simulink model "HIWIN_arm-DESKTOP-VMBR1O2"  (R2022b)
settings: Solver=ode4  StartTime=0  StopTime=1.4435  FixedStep=0.0005  RelTol=1e-3
model workspace (MAT data in the model file):
  Link1_init = 0
  Link2_init = 0
  Link3_init = 0
  Link4_init = 0
  Link5_init = 0
  Link6_init = 0
values from neighbouring files (symbols this model uses):
  b1 = evalin('base','b1')    [Freq_response.m]    (also in Parameters.m = B(1); parameters.mat = 38.5729006482)
  b2 = evalin('base','b2')    [Freq_response.m]    (also in Parameters.m = B(2); parameters.mat = 28.585362141)
  b3 = evalin('base','b3')    [Freq_response.m]    (also in Parameters.m = B(3); parameters.mat = 10.962587304)
  b4 = evalin('base','b4')    [Freq_response.m]    (also in Parameters.m = B(4); parameters.mat = 5.56110095294)
  b5 = evalin('base','b5')    [Freq_response.m]    (also in Parameters.m = B(5); parameters.mat = 1.70954720068)
  b6 = evalin('base','b6')    [Freq_response.m]    (also in Parameters.m = B(6); parameters.mat = 1.09956377442)
  J1 = evalin('base','J1')    [Freq_response.m]    (also in Parameters.m = 2.390528; parameters.mat = 2.390528)
  J2 = evalin('base','J2')    [Freq_response.m]    (also in Parameters.m = 3.0413; parameters.mat = 3.0413)
  J3 = evalin('base','J3')    [Freq_response.m]    (also in Parameters.m = 0.716992; parameters.mat = 0.716992)
  J4 = evalin('base','J4')    [Freq_response.m]    (also in Parameters.m = 0.37850409; parameters.mat = 0.37850409)
  J5 = evalin('base','J5')    [Freq_response.m]    (also in Parameters.m = 0.076544; parameters.mat = 0.076544)
  J6 = evalin('base','J6')    [Freq_response.m]    (also in Parameters.m = 0.03665; parameters.mat = 0.03665)
  Kt1 = evalin('base','Kt1')    [Freq_response.m]    (also in Parameters.m = 0.524; parameters.mat = 0.524)
  Kt2 = evalin('base','Kt2')    [Freq_response.m]    (also in Parameters.m = 0.524; parameters.mat = 0.524)
  Kt3 = evalin('base','Kt3')    [Freq_response.m]    (also in Parameters.m = 0.476; parameters.mat = 0.476)
  Kt4 = evalin('base','Kt4')    [Freq_response.m]    (also in Parameters.m = 0.424; parameters.mat = 0.424)
  Kt5 = evalin('base','Kt5')    [Freq_response.m]    (also in Parameters.m = 0.246; parameters.mat = 0.246)
  Kt6 = evalin('base','Kt6')    [Freq_response.m]    (also in Parameters.m = 0.246; parameters.mat = 0.246)
libraries: slpidlib x38
(part 4 of 4)

== system HIWIN_arm-DESKTOP-VMBR1O2/link test/link6 ==
  In2 : Inport
  In1 : Inport  Port=2
  Integrator : Integrator
  Kp : slpidlib/PID Controller  Controller=PI  Form=Ideal  TimeDomain=Continuous-time  UseExternalTs=off  SampleTime=-1  IntegratorMethod=Forward Euler  FilterMethod=Forward Euler  ControllerParametersSource=internal  P=105.919532331885  I=2.29576855307102  UseKiTs=off  D=0  N=100  UseFilter=on  TunerSelectOption=Transfer Function Based (PID Tuner App)  InitialConditionSource=internal  InitialConditionForIntegrator=0  InitialConditionForFilter=0  DifferentiatorICPrevScaledInput=0  ExternalReset=none  TrackingMode=off  Kt=1  LimitOutput=off  SatLimitsSource=internal  UpperSaturationLimit=inf  LowerSaturationLimit=-inf  LinearizeAsGain=on  AntiWindupMode=none  Kb=1  LimitIntegrator=off  UpperIntegratorSaturationLimit=inf  LowerIntegratorSaturationLimit=-inf  POutMin=[]  POutMax=[]  IOutMin=[]  IOutMax=[]  DOutMin=[]  DOutMax=[]  NOutMin=[]  NOutMax=[]  SumOutMin=[]  SumOutMax=[]  SaturationOutMin=[]  SaturationOutMax=[]  PParamMin=[]  PParamMax=[]  IParamMin=[]  IParamMax=[]  DParamMin=[]  DParamMax=[]  NParamMin=[]  NParamMax=[]  KbParamMin=[]  KbParamMax=[]  KtParamMin=[]  KtParamMax=[]  KbOutMin=[]  KbOutMax=[]  KtOutMin=[]  KtOutMax=[]  IntegratorOutMin=[]  IntegratorOutMax=[]  FilterOutMin=[]  FilterOutMax=[]  SumI1OutMin=[]  SumI1OutMax=[]  SumI2OutMin=[]  SumI2OutMax=[]  SumI3OutMin=[]  SumI3OutMax=[]  SumI4OutMin=[]  SumI4OutMax=[]  SumDOutMin=[]  SumDOutMax=[]  DifferentiatorOutMin=[]  DifferentiatorOutMax=[]  FilterDiffOutCoefMin=[]  FilterDiffOutCoefMax=[]  ReciprocalOutMin=[]  ReciprocalOutMax=[]  SumDenOutMin=[]  SumDenOutMax=[]  SumNumOutMin=[]  SumNumOutMax=[]  DivideOutMin=[]  DivideOutMax=[]  UdiffTsProdOutMin=[]  UdiffTsProdOutMax=[]  NTsProdOutMin=[]  NTsProdOutMax=[]  UintegralTsProdOutMin=[]  UintegralTsProdOutMax=[]  UngainTsProdOutMin=[]  UngainTsProdOutMax=[]  ClampingZeroOutDataTypeStr=Inherit: Inherit via back propagation  ClampingZeroOutMin=[]  ClampingZeroOutMax=[]  FilterDenConstantOutDataTypeStr=Inherit: Inherit via back propagation  FilterDenConstantOutMin=[]  FilterDenConstantOutMax=[]  PCopyOutDataTypeStr=Inherit: Inherit via back propagation  PCopyOutMin=[]  PCopyOutMax=[]  NCopyOutDataTypeStr=Inherit: Inherit via back propagation  NCopyOutMin=[]  NCopyOutMax=[]  IntegratorContinuousStateAttributes=''  IntegratorStateMustResolveToSignalObject=off  IntegratorRTWStateStorageClass=Auto  FilterContinuousStateAttributes=''  FilterStateMustResolveToSignalObject=off  FilterRTWStateStorageClass=Auto  ParallelPVariant=Passthrough  IdealPVariant=InternalParameters  IVariant=InternalParameters  DVariant=Disabled  IntegratorVariant=Continuous  SatVariant=Disabled  AWVariant=Passthrough  PCopyVariant=Disabled  TRVariant=Disabled  FdbkBlocksVariant=Forward  IdealPFdbkVariant=Disabled  SatFdbkVariant=Disabled  DerivativeFilterVariant=Disabled  NVariant=Disabled  NCopyVariant=Disabled_SignalSpec  FilterICVariant=Disabled  IntegratorICVariant=InternalICs  ExternalResetVariant=Disabled  TRSumVariant=Passthrough  SumFdbkVariant=Disabled  SumVariant=Sum_PI  TsampFilterVariant=InternalTs  TsampNgainVariant=Passthrough  TsampIntegralVariant=Passthrough  ExternalSaturationOutDataTypeStr=Inherit: Same as second input
  Kt : Gain  Gain=Kt6
  Kv : slpidlib/PID Controller  Controller=PI  Form=Ideal  TimeDomain=Continuous-time  UseExternalTs=off  SampleTime=-1  IntegratorMethod=Forward Euler  FilterMethod=Forward Euler  ControllerParametersSource=internal  P=21.6698338640267  I=151.095812250567  UseKiTs=off  D=0  N=100  UseFilter=on  TunerSelectOption=Transfer Function Based (PID Tuner App)  InitialConditionSource=internal  InitialConditionForIntegrator=0  InitialConditionForFilter=0  DifferentiatorICPrevScaledInput=0  ExternalReset=none  TrackingMode=off  Kt=1  LimitOutput=off  SatLimitsSource=internal  UpperSaturationLimit=inf  LowerSaturationLimit=-inf  LinearizeAsGain=on  AntiWindupMode=none  Kb=1  LimitIntegrator=off  UpperIntegratorSaturationLimit=inf  LowerIntegratorSaturationLimit=-inf  POutMin=[]  POutMax=[]  IOutMin=[]  IOutMax=[]  DOutMin=[]  DOutMax=[]  NOutMin=[]  NOutMax=[]  SumOutMin=[]  SumOutMax=[]  SaturationOutMin=[]  SaturationOutMax=[]  PParamMin=[]  PParamMax=[]  IParamMin=[]  IParamMax=[]  DParamMin=[]  DParamMax=[]  NParamMin=[]  NParamMax=[]  KbParamMin=[]  KbParamMax=[]  KtParamMin=[]  KtParamMax=[]  KbOutMin=[]  KbOutMax=[]  KtOutMin=[]  KtOutMax=[]  IntegratorOutMin=[]  IntegratorOutMax=[]  FilterOutMin=[]  FilterOutMax=[]  SumI1OutMin=[]  SumI1OutMax=[]  SumI2OutMin=[]  SumI2OutMax=[]  SumI3OutMin=[]  SumI3OutMax=[]  SumI4OutMin=[]  SumI4OutMax=[]  SumDOutMin=[]  SumDOutMax=[]  DifferentiatorOutMin=[]  DifferentiatorOutMax=[]  FilterDiffOutCoefMin=[]  FilterDiffOutCoefMax=[]  ReciprocalOutMin=[]  ReciprocalOutMax=[]  SumDenOutMin=[]  SumDenOutMax=[]  SumNumOutMin=[]  SumNumOutMax=[]  DivideOutMin=[]  DivideOutMax=[]  UdiffTsProdOutMin=[]  UdiffTsProdOutMax=[]  NTsProdOutMin=[]  NTsProdOutMax=[]  UintegralTsProdOutMin=[]  UintegralTsProdOutMax=[]  UngainTsProdOutMin=[]  UngainTsProdOutMax=[]  ClampingZeroOutDataTypeStr=Inherit: Inherit via back propagation  ClampingZeroOutMin=[]  ClampingZeroOutMax=[]  FilterDenConstantOutDataTypeStr=Inherit: Inherit via back propagation  FilterDenConstantOutMin=[]  FilterDenConstantOutMax=[]  PCopyOutDataTypeStr=Inherit: Inherit via back propagation  PCopyOutMin=[]  PCopyOutMax=[]  NCopyOutDataTypeStr=Inherit: Inherit via back propagation  NCopyOutMin=[]  NCopyOutMax=[]  IntegratorContinuousStateAttributes=''  IntegratorStateMustResolveToSignalObject=off  IntegratorRTWStateStorageClass=Auto  FilterContinuousStateAttributes=''  FilterStateMustResolveToSignalObject=off  FilterRTWStateStorageClass=Auto  ParallelPVariant=Passthrough  IdealPVariant=InternalParameters  IVariant=InternalParameters  DVariant=Disabled  IntegratorVariant=Continuous  SatVariant=Disabled  AWVariant=Passthrough  PCopyVariant=Disabled  TRVariant=Disabled  FdbkBlocksVariant=Forward  IdealPFdbkVariant=Disabled  SatFdbkVariant=Disabled  DerivativeFilterVariant=Disabled  NVariant=Disabled  NCopyVariant=Disabled_SignalSpec  FilterICVariant=Disabled  IntegratorICVariant=InternalICs  ExternalResetVariant=Disabled  TRSumVariant=Passthrough  SumFdbkVariant=Disabled  SumVariant=Sum_PI  TsampFilterVariant=InternalTs  TsampNgainVariant=Passthrough  TsampIntegralVariant=Passthrough  ExternalSaturationOutDataTypeStr=Inherit: Same as second input
  Sum2 : Sum  Inputs=|+-
  Sum3 : Sum  Inputs=|+-
  Sum4 : Sum  Inputs=|+-
  Transfer Fcn1 : TransferFcn  Denominator=[J6 b6]
  theta : Outport
  wires:
  Sum2/1 -> Kv/1
  Transfer Fcn1/1 -> Integrator/1, Sum2/2  "theta dot"
  Kv/1 -> Kt/1
  Kt/1 -> Sum4/1  "T"
  Sum4/1 -> Transfer Fcn1/1
  In2/1 -> Sum4/2
  Sum3/1 -> Kp/1
  Kp/1 -> Sum2/1
  In1/1 -> Sum3/1
  Integrator/1 -> Sum3/2, theta/1

== system HIWIN_arm-DESKTOP-VMBR1O2/link test/link6_test ==
  In1 : Inport
  Integrator : Integrator
  Kp : slpidlib/PID Controller  Controller=PI  Form=Ideal  TimeDomain=Continuous-time  UseExternalTs=off  SampleTime=-1  IntegratorMethod=Forward Euler  FilterMethod=Forward Euler  ControllerParametersSource=internal  P=5.27011747503354  I=0.0922424275458122  UseKiTs=off  D=0  N=100  UseFilter=on  TunerSelectOption=Transfer Function Based (PID Tuner App)  InitialConditionSource=internal  InitialConditionForIntegrator=0  InitialConditionForFilter=0  DifferentiatorICPrevScaledInput=0  ExternalReset=none  TrackingMode=off  Kt=1  LimitOutput=off  SatLimitsSource=internal  UpperSaturationLimit=inf  LowerSaturationLimit=-inf  LinearizeAsGain=on  AntiWindupMode=none  Kb=1  LimitIntegrator=off  UpperIntegratorSaturationLimit=inf  LowerIntegratorSaturationLimit=-inf  POutMin=[]  POutMax=[]  IOutMin=[]  IOutMax=[]  DOutMin=[]  DOutMax=[]  NOutMin=[]  NOutMax=[]  SumOutMin=[]  SumOutMax=[]  SaturationOutMin=[]  SaturationOutMax=[]  PParamMin=[]  PParamMax=[]  IParamMin=[]  IParamMax=[]  DParamMin=[]  DParamMax=[]  NParamMin=[]  NParamMax=[]  KbParamMin=[]  KbParamMax=[]  KtParamMin=[]  KtParamMax=[]  KbOutMin=[]  KbOutMax=[]  KtOutMin=[]  KtOutMax=[]  IntegratorOutMin=[]  IntegratorOutMax=[]  FilterOutMin=[]  FilterOutMax=[]  SumI1OutMin=[]  SumI1OutMax=[]  SumI2OutMin=[]  SumI2OutMax=[]  SumI3OutMin=[]  SumI3OutMax=[]  SumI4OutMin=[]  SumI4OutMax=[]  SumDOutMin=[]  SumDOutMax=[]  DifferentiatorOutMin=[]  DifferentiatorOutMax=[]  FilterDiffOutCoefMin=[]  FilterDiffOutCoefMax=[]  ReciprocalOutMin=[]  ReciprocalOutMax=[]  SumDenOutMin=[]  SumDenOutMax=[]  SumNumOutMin=[]  SumNumOutMax=[]  DivideOutMin=[]  DivideOutMax=[]  UdiffTsProdOutMin=[]  UdiffTsProdOutMax=[]  NTsProdOutMin=[]  NTsProdOutMax=[]  UintegralTsProdOutMin=[]  UintegralTsProdOutMax=[]  UngainTsProdOutMin=[]  UngainTsProdOutMax=[]  ClampingZeroOutDataTypeStr=Inherit: Inherit via back propagation  ClampingZeroOutMin=[]  ClampingZeroOutMax=[]  FilterDenConstantOutDataTypeStr=Inherit: Inherit via back propagation  FilterDenConstantOutMin=[]  FilterDenConstantOutMax=[]  PCopyOutDataTypeStr=Inherit: Inherit via back propagation  PCopyOutMin=[]  PCopyOutMax=[]  NCopyOutDataTypeStr=Inherit: Inherit via back propagation  NCopyOutMin=[]  NCopyOutMax=[]  IntegratorContinuousStateAttributes=''  IntegratorStateMustResolveToSignalObject=off  IntegratorRTWStateStorageClass=Auto  FilterContinuousStateAttributes=''  FilterStateMustResolveToSignalObject=off  FilterRTWStateStorageClass=Auto  ParallelPVariant=Passthrough  IdealPVariant=InternalParameters  IVariant=InternalParameters  DVariant=Disabled  IntegratorVariant=Continuous  SatVariant=Disabled  AWVariant=Passthrough  PCopyVariant=Disabled  TRVariant=Disabled  FdbkBlocksVariant=Forward  IdealPFdbkVariant=Disabled  SatFdbkVariant=Disabled  DerivativeFilterVariant=Disabled  NVariant=Disabled  NCopyVariant=Disabled_SignalSpec  FilterICVariant=Disabled  IntegratorICVariant=InternalICs  ExternalResetVariant=Disabled  TRSumVariant=Passthrough  SumFdbkVariant=Disabled  SumVariant=Sum_PI  TsampFilterVariant=InternalTs  TsampNgainVariant=Passthrough  TsampIntegralVariant=Passthrough  ExternalSaturationOutDataTypeStr=Inherit: Same as second input
  Kt : Gain  Gain=Kt6
  Kv : slpidlib/PID Controller  Controller=PI  Form=Ideal  TimeDomain=Continuous-time  UseExternalTs=off  SampleTime=-1  IntegratorMethod=Forward Euler  FilterMethod=Forward Euler  ControllerParametersSource=internal  P=8.61933922965824e-06  I=187982.02415467  UseKiTs=off  D=0  N=100  UseFilter=on  TunerSelectOption=Transfer Function Based (PID Tuner App)  InitialConditionSource=internal  InitialConditionForIntegrator=0  InitialConditionForFilter=0  DifferentiatorICPrevScaledInput=0  ExternalReset=none  TrackingMode=off  Kt=1  LimitOutput=off  SatLimitsSource=internal  UpperSaturationLimit=inf  LowerSaturationLimit=-inf  LinearizeAsGain=on  AntiWindupMode=none  Kb=1  LimitIntegrator=off  UpperIntegratorSaturationLimit=inf  LowerIntegratorSaturationLimit=-inf  POutMin=[]  POutMax=[]  IOutMin=[]  IOutMax=[]  DOutMin=[]  DOutMax=[]  NOutMin=[]  NOutMax=[]  SumOutMin=[]  SumOutMax=[]  SaturationOutMin=[]  SaturationOutMax=[]  PParamMin=[]  PParamMax=[]  IParamMin=[]  IParamMax=[]  DParamMin=[]  DParamMax=[]  NParamMin=[]  NParamMax=[]  KbParamMin=[]  KbParamMax=[]  KtParamMin=[]  KtParamMax=[]  KbOutMin=[]  KbOutMax=[]  KtOutMin=[]  KtOutMax=[]  IntegratorOutMin=[]  IntegratorOutMax=[]  FilterOutMin=[]  FilterOutMax=[]  SumI1OutMin=[]  SumI1OutMax=[]  SumI2OutMin=[]  SumI2OutMax=[]  SumI3OutMin=[]  SumI3OutMax=[]  SumI4OutMin=[]  SumI4OutMax=[]  SumDOutMin=[]  SumDOutMax=[]  DifferentiatorOutMin=[]  DifferentiatorOutMax=[]  FilterDiffOutCoefMin=[]  FilterDiffOutCoefMax=[]  ReciprocalOutMin=[]  ReciprocalOutMax=[]  SumDenOutMin=[]  SumDenOutMax=[]  SumNumOutMin=[]  SumNumOutMax=[]  DivideOutMin=[]  DivideOutMax=[]  UdiffTsProdOutMin=[]  UdiffTsProdOutMax=[]  NTsProdOutMin=[]  NTsProdOutMax=[]  UintegralTsProdOutMin=[]  UintegralTsProdOutMax=[]  UngainTsProdOutMin=[]  UngainTsProdOutMax=[]  ClampingZeroOutDataTypeStr=Inherit: Inherit via back propagation  ClampingZeroOutMin=[]  ClampingZeroOutMax=[]  FilterDenConstantOutDataTypeStr=Inherit: Inherit via back propagation  FilterDenConstantOutMin=[]  FilterDenConstantOutMax=[]  PCopyOutDataTypeStr=Inherit: Inherit via back propagation  PCopyOutMin=[]  PCopyOutMax=[]  NCopyOutDataTypeStr=Inherit: Inherit via back propagation  NCopyOutMin=[]  NCopyOutMax=[]  IntegratorContinuousStateAttributes=''  IntegratorStateMustResolveToSignalObject=off  IntegratorRTWStateStorageClass=Auto  FilterContinuousStateAttributes=''  FilterStateMustResolveToSignalObject=off  FilterRTWStateStorageClass=Auto  ParallelPVariant=Passthrough  IdealPVariant=InternalParameters  IVariant=InternalParameters  DVariant=Disabled  IntegratorVariant=Continuous  SatVariant=Disabled  AWVariant=Passthrough  PCopyVariant=Disabled  TRVariant=Disabled  FdbkBlocksVariant=Forward  IdealPFdbkVariant=Disabled  SatFdbkVariant=Disabled  DerivativeFilterVariant=Disabled  NVariant=Disabled  NCopyVariant=Disabled_SignalSpec  FilterICVariant=Disabled  IntegratorICVariant=InternalICs  ExternalResetVariant=Disabled  TRSumVariant=Passthrough  SumFdbkVariant=Disabled  SumVariant=Sum_PI  TsampFilterVariant=InternalTs  TsampNgainVariant=Passthrough  TsampIntegralVariant=Passthrough  ExternalSaturationOutDataTypeStr=Inherit: Same as second input
  Scope : Scope
  Sum2 : Sum  Inputs=|+-
  Sum3 : Sum  Inputs=|+-
  Transfer Fcn1 : TransferFcn  Denominator=[J6 b6]
  theta : Outport
  wires:
  In1/1 -> Sum3/1
  Kp/1 -> Sum2/1
  Sum3/1 -> Kp/1
  Integrator/1 -> theta/1, Scope/1, Sum3/2  "theta dot"
  Sum2/1 -> Kv/1
  Kt/1 -> Transfer Fcn1/1  "T"
  Transfer Fcn1/1 -> Sum2/2, Integrator/1  "theta dot"
  Kv/1 -> Kt/1

== matlab function HIWIN_arm-DESKTOP-VMBR1O2/Forwar kinematic ==
  data: q1 input; X output; q2 input; q3 input; q4 input; q5 input; q6 input; Y output; Z output
function [X, Y, Z] = RT605_FK_Mat(q1, q2, q3, q4, q5, q6)
% T = [0;0;120];
T = [0;0;120];
% T = [xtool; ytool; ztool]
%RT605_FK
%    T07 = RT605_FK(Q1,Q2,Q3,Q4,Q5,Q6)

%    This function was generated by the Symbolic Math Toolbox version 8.1.
%    17-Nov-2020 11:11:13
q1 = deg2rad(q1);
q2 = deg2rad(q2);
q3 = deg2rad(q3);
q4 = deg2rad(q4);
q5 = deg2rad(q5);
q6 = deg2rad(q6);

t2 = cos(q1);
t3 = sin(q1);
t4 = sin(q4);
t5 = cos(q4);
t6 = cos(q2);
t7 = cos(q3);
t8 = sin(q2);
t9 = sin(q3);
t13 = t2.*t6.*t7;
t14 = t2.*t8.*t9;
t10 = t13-t14;
t11 = cos(q6);
t12 = t3.*t5;
t15 = t12-t4.*t10;
t16 = sin(q6);
t17 = cos(q5);
t18 = t3.*t4;
t19 = t5.*t10;
t20 = t18+t19;
t21 = sin(q5);
t22 = t2.*t6.*t9;
t23 = t2.*t7.*t8;
t24 = t22+t23;
t25 = t17.*t20-t21.*t24;
t26 = t3.*t6.*t7;
t29 = t3.*t8.*t9;
t27 = t26-t29;
t28 = t2.*t5;
t30 = t4.*t27;
t31 = t28+t30;
t32 = t2.*t4;
t40 = t5.*t27;
t33 = t32-t40;
t34 = t17.*t33;
t35 = t3.*t6.*t9;
t36 = t3.*t7.*t8;
t37 = t35+t36;
t38 = t21.*t37;
t39 = t34+t38;
t41 = q2+q3;
t42 = sin(t41);
t43 = cos(t41);
t44 = t21.*t43;
t45 = t5.*t17.*t42;
t46 = t44+t45;
T07 = reshape([t15.*t16+t11.*t25,-t16.*t31-t11.*t39,t11.*t46-t4.*t16.*t42,0.0,t11.*t15-t16.*t25,-t11.*t31+t16.*t39,-t16.*t46-t4.*t11.*t42,0.0,t17.*t24+t20.*t21,t17.*t37-t21.*t33,-t17.*t43+t5.*t21.*t42,0.0,t2.*3.0e1+t2.*t6.*3.4e2+t2.*t6.*t7.*4.0e1+t2.*t6.*t9.*3.38e2+t2.*t7.*t8.*3.38e2-t2.*t8.*t9.*4.0e1+t3.*t4.*t21.*(1.73e2./2.0)+t2.*t17.*t42.*(1.73e2./2.0)+t2.*t5.*t6.*t7.*t21.*(1.73e2./2.0)-t2.*t5.*t8.*t9.*t21.*(1.73e2./2.0),t3.*3.0e1+t3.*t6.*3.4e2+t3.*t6.*t7.*4.0e1+t3.*t6.*t9.*3.38e2+t3.*t7.*t8.*3.38e2-t3.*t8.*t9.*4.0e1-t2.*t4.*t21.*(1.73e2./2.0)+t3.*t17.*t42.*(1.73e2./2.0)+t3.*t5.*t6.*t7.*t21.*(1.73e2./2.0)-t3.*t5.*t8.*t9.*t21.*(1.73e2./2.0),t8.*3.4e2+t42.*4.0e1-t43.*3.38e2-t17.*t43.*(1.73e2./2.0)+t42.*sin(q4+q5).*(1.73e2./4.0)-t42.*sin(q4-q5).*(1.73e2./4.0),1.0],[4,4]);
T07 = T07*[eye(3), T; [0, 0, 0, 1]];
% 把長度單位換成 m

T07(1:3, 4) = T07(1:3, 4)/1000;

X = T07(1,4);
Y = T07(2,4);
Z = T07(3,4);

== matlab function HIWIN_arm-DESKTOP-VMBR1O2/MATLAB Function ==
  data: tor1 output; tor2 output; tor3 output; tor4 output; tor5 output; q2 input; q3 input; q4 input; q5 input; q6 input; tor6 output; mode input
function [tor1,       tor2,       tor3,       tor4,       tor5,       tor6]       = computeRT605_GTorque(q2, q3, q4,q5,q6, mode)

   if mode==1
    % Joint space (unit: N-m)
    % Joint unit: rad
    m2=8.663838679819902;
    m3=3.666344308215677;
    m4=3.615885748802093;
    m5= 1.030957155800785;
    m6= 1.516126236073167;
    rcx2 = -0.144212674049077;
    rcy2 = 0.030223509965502;


    rcx3 = -0.033723402680331;
    rcz3 = 0.052721699263344;

    rcx4 = -0.001489966345731;
    rcy4 = 0.156987050585444;
    rcz4 =-0.001747720466200;

    rcx5 = -0.005033704747790;
    rcy5 = -0.001191062175159;
    rcz5 = 0.074853989870876;

    rcx6 = 8.855201349532231e-04;
    rcy6 = -2.306859519121158e-04;
    rcz6 =0.045616506355611;

    t2 = cos(q2);
    t3 = cos(q4);
    t4 = cos(q5);
    t5 = cos(q6);
    t6 = sin(q4);
    t7 = sin(q5);
    t8 = sin(q6);
    t9 = q2+q3;
    t10 = q4+q5;
    t11 = q4+q6;
    t16 = -q5;
    t17 = -q6;
    t12 = cos(t9);
    t13 = cos(t10);
    t14 = sin(t9);
    t15 = sin(t10);
    t18 = q4+t16;
    t19 = q4+t17;
    t20 = cos(t18);
    t21 = sin(t18);
    t22 = m3.*t12.*3.924e-1;
    t23 = m4.*t12.*3.924e-1;
    t24 = m5.*t12.*3.924e-1;
    t25 = m6.*t12.*3.924e-1;
    t26 = m3.*rcx3.*t12.*(9.81e+2./1.0e+2);
    t27 = m4.*rcy4.*t14.*(9.81e+2./1.0e+2);
    t28 = m3.*rcz3.*t14.*(9.81e+2./1.0e+2);
    t30 = m4.*rcx4.*t3.*t12.*(9.81e+2./1.0e+2);
    t31 = m5.*rcy5.*t6.*t12.*(9.81e+2./1.0e+2);
    t32 = m4.*rcz4.*t6.*t12.*(9.81e+2./1.0e+2);
    t33 = m5.*rcz5.*t4.*t14.*(9.81e+2./1.0e+2);
    t34 = m6.*rcz6.*t4.*t14.*(9.81e+2./1.0e+2);
    t35 = m5.*rcx5.*t7.*t14.*(9.81e+2./1.0e+2);
    t36 = m4.*t14.*3.31578;
    t37 = m5.*t14.*3.31578;
    t38 = m6.*t14.*3.31578;
    t42 = m6.*rcx6.*t5.*t7.*t14.*(9.81e+2./1.0e+2);
    t43 = m6.*rcy6.*t7.*t8.*t14.*(9.81e+2./1.0e+2);
    t45 = m6.*t4.*t14.*8.48565e-1;
    t29 = -t27;
    t39 = -t31;
    t40 = -t32;
    t41 = -t35;
    t44 = -t42;
    G = [zeros(1, length(t44));t22+t23+t24+t25+t26+t28+t29+t30+t33+t34+t36+t37+t38+t39+t40+t41+t43+t44+t45+m2.*t2.*3.3354+m3.*t2.*3.3354+m4.*t2.*3.3354+m5.*t2.*3.3354+m6.*t2.*3.3354-m2.*rcy2.*sin(q2).*(9.81e+2./1.0e+2)+m2.*rcx2.*t2.*(9.81e+2./1.0e+2)+m6.*t12.*t15.*4.242825e-1-m6.*t12.*t21.*4.242825e-1+m5.*rcx5.*t12.*t13.*(9.81e+2./2.0e+2)+m5.*rcx5.*t12.*t20.*(9.81e+2./2.0e+2)+m5.*rcz5.*t12.*t15.*(9.81e+2./2.0e+2)+m6.*rcz6.*t12.*t15.*(9.81e+2./2.0e+2)-m5.*rcz5.*t12.*t21.*(9.81e+2./2.0e+2)-m6.*rcz6.*t12.*t21.*(9.81e+2./2.0e+2)+m6.*rcx6.*t12.*cos(t11).*(9.81e+2./2.0e+2)-m6.*rcx6.*t12.*cos(t19).*(9.81e+2./2.0e+2)-m6.*rcy6.*t12.*sin(t11).*(9.81e+2./2.0e+2)-m6.*rcy6.*t12.*sin(t19).*(9.81e+2./2.0e+2)+m6.*rcx6.*t5.*t12.*t13.*(9.81e+2./2.0e+2)+m6.*rcx6.*t5.*t12.*t20.*(9.81e+2./2.0e+2)-m6.*rcy6.*t8.*t12.*t13.*(9.81e+2./2.0e+2)-m6.*rcy6.*t8.*t12.*t20.*(9.81e+2./2.0e+2);t22+t23+t24+t25+t26+t28+t29+t30+t33+t34+t36+t37+t38+t39+t40+t41+t43+t44+t45+m6.*t3.*t7.*t12.*8.48565e-1+m5.*rcx5.*t3.*t4.*t12.*(9.81e+2./1.0e+2)-m6.*rcx6.*t6.*t8.*t12.*(9.81e+2./1.0e+2)-m6.*rcy6.*t5.*t6.*t12.*(9.81e+2./1.0e+2)+m5.*rcz5.*t3.*t7.*t12.*(9.81e+2./1.0e+2)+m6.*rcz6.*t3.*t7.*t12.*(9.81e+2./1.0e+2)+m6.*rcx6.*t3.*t4.*t5.*t12.*(9.81e+2./1.0e+2)-m6.*rcy6.*t3.*t4.*t8.*t12.*(9.81e+2./1.0e+2);t14.*(m4.*rcx4.*t6.*2.0e+3+m5.*rcy5.*t3.*2.0e+3+m4.*rcz4.*t3.*2.0e+3+m6.*t6.*t7.*1.73e+2+m5.*rcx5.*t4.*t6.*2.0e+3+m6.*rcx6.*t3.*t8.*2.0e+3+m6.*rcy6.*t3.*t5.*2.0e+3+m5.*rcz5.*t6.*t7.*2.0e+3+m6.*rcz6.*t6.*t7.*2.0e+3+m6.*rcx6.*t4.*t5.*t6.*2.0e+3-m6.*rcy6.*t4.*t6.*t8.*2.0e+3).*(-4.905e-3);m6.*(t7.*t12.*8.65e-2+rcz6.*t7.*t12+t3.*t4.*t14.*8.65e-2+rcx6.*t4.*t5.*t12-rcy6.*t4.*t8.*t12+rcz6.*t3.*t4.*t14-rcx6.*t3.*t5.*t7.*t14+rcy6.*t3.*t7.*t8.*t14).*(9.81e+2./1.0e+2)+m5.*(rcx5.*t4.*t12+rcz5.*t7.*t12-rcx5.*t3.*t7.*t14+rcz5.*t3.*t4.*t14).*(9.81e+2./1.0e+2);m6.*(rcx6.*(t5.*t6.*t14+t7.*t8.*t12+t3.*t4.*t8.*t14)+rcy6.*(t5.*t7.*t12-t6.*t8.*t14+t3.*t4.*t5.*t14)).*(-9.81e+2./1.0e+2)];
       
    tor = G';
    tor1 = tor(1);
    tor2 = tor(2);
    tor3 = tor(3);
    tor4 = tor(4);
    tor5 = tor(5);
    tor6 = tor(6);
   else
       tor1 = 0;
       tor2 = 0;
       tor3 = 0;
       tor4 = 0;
       tor5 = 0;
       tor6 = 0;
   end
end

== matlab function HIWIN_arm-DESKTOP-VMBR1O2/inverse Kinematic ==
  data: px input; py input; pz input; Theta1 output; Theta2 output; Theta3 output
function [Theta1,Theta2, Theta3] = Inverse(px,py,pz)

a1=0.03;
a2=0.34;
a3=0.04;
d4=0.338;

Theta1 = atan2(py,px); % 

G1 = px*cos(Theta1) + py*sin(Theta1);
k1 = ((G1-a1)*(G1-a1) + pz*pz - a2*a2 - a3*a3 - d4*d4)/2*a2;
phi = atan2(a3, d4);
lo = sqrt(a3*a3 + d4*d4);

Theta3 = atan2(a3, d4) - atan2(k1, sqrt(lo/lo - k1*k1)); %sqrt(lo/lo - k1*k1)

Theta2 = atan2((G1-a1)*(-d4+a2*sin(Theta3) - pz*(a3+a2*cos(Theta3))) , ...
               (G1-a1)*(a3+a2*cos(Theta3) + pz*(-d4+a2*sin(Theta3)))) - Theta3;

end
